simulink model "Ass2_Full"  (R2024b)
settings: Solver=VariableStepAuto  StartTime=0.0  StopTime=0.3  MaxStep=1e-5  RelTol=1e-4
values from neighbouring files (symbols this model uses):
  Cdc = 2*tau_C*Sn_n1/Vdcref_n1^2    (= 0.277777777778)    [PMSG_B2B_init.m]
  Rs = 0.01    [PMSG_B2B_init.m]
undefined symbols (not defined in the file or in its folder): a, f, G, Gn, Gstep, idref, iqref, Isc, Ki, kic, kip, kiv, kpc, kpp, kpv, Kv, L, Lg, par, Pref, Qref, Rc, Rg, Rp, ser, T, Tn, Tstep, Vdc_ref, Voc, Vpeak, Vt
libraries: spsControlledVoltageSourceLib x6, slpidlib x6, spsVoltageMeasurementLib x4, spsControlledCurrentSourceLib x2, spsThreePhaseSeriesRLCBranchLib x2, spsCurrentMeasurementLib x2, spsGroundLib x2, spsThreePhaseVIMeasurementLib x1, spsSeriesRLCBranchLib x1, sps_lib x1
settings Model: Creator=sproj  LastModifiedBy=sproj

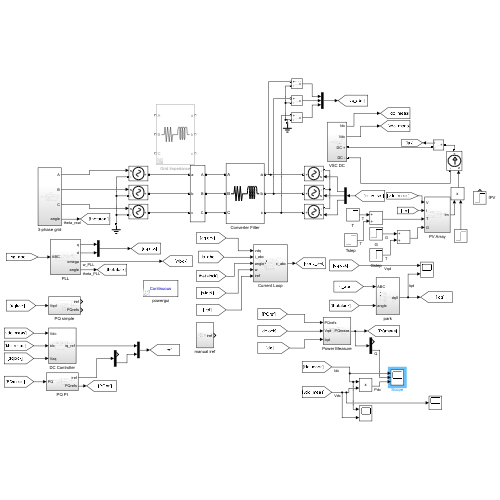
[thumbnail: Simulink's stored preview of the top-level diagram]
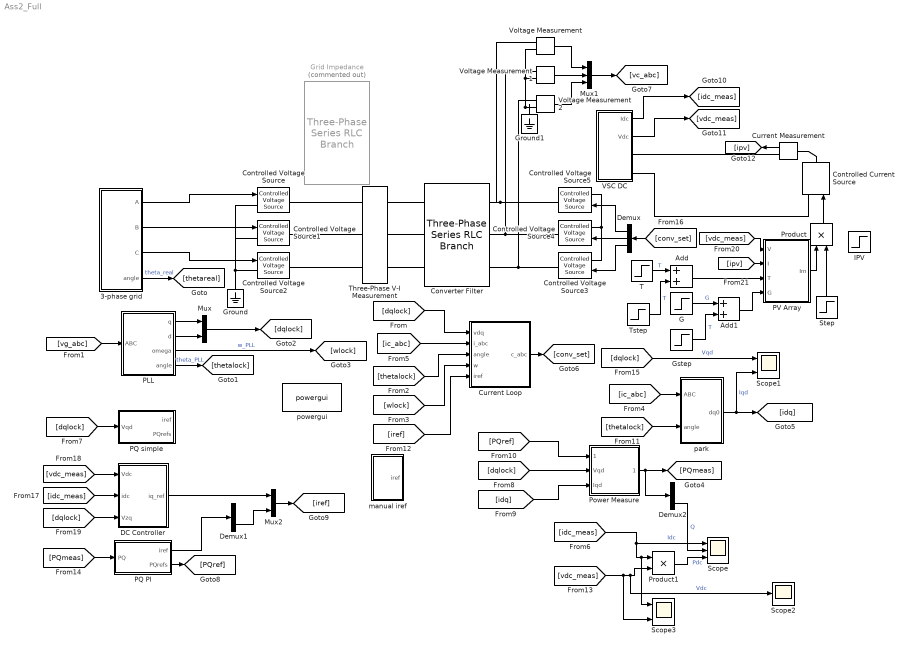
== system Ass2_Full ==
  3-phase grid : Subsystem
  Add : Sum
  Add1 : Sum
  Controlled Current Source : spsControlledCurrentSourceLib/Controlled Current Source  Initialize=on  Source_Type=AC  Amplitude=0  Phase=0  Frequency=0  Measurements=None
  Controlled Voltage Source{,1..5} (6 alike) : spsControlledVoltageSourceLib/Controlled Voltage Source  Initialize=on  Source_Type=AC  Amplitude=0  Phase=0  Frequency=0  Measurements=None
  Converter Filter : spsThreePhaseSeriesRLCBranchLib/Three-Phase Series RLC Branch  LConnTagsString=A|B|C  RConnTagsString=A|B|C  BranchType=RL  Resistance=Rc  Inductance=L  Capacitance=1e-6  Measurements=None
  Current Loop : Subsystem
  Current Measurement : spsCurrentMeasurementLib/Current Measurement  PhasorSimulation=off  OutputType=Complex  PSBequivalent=0
  DC Controller : Subsystem
  Demux : Demux  Outputs=3
  Demux1 : Demux  Outputs=2
  Demux2 : Demux  Outputs=2
  G : Step  Time=0  After=G  SampleTime=0
  Grid Impedance : spsThreePhaseSeriesRLCBranchLib/Three-Phase Series RLC Branch  Commented=on  LConnTagsString=A|B|C  RConnTagsString=A|B|C  BranchType=RL  Resistance=Rg  Inductance=Lg  Capacitance=1e-6  Measurements=None
  Ground : spsGroundLib/Ground  LConnTagsString=a
  Ground1 : spsGroundLib/Ground  LConnTagsString=a
  Gstep : Step  Time=0.05  After=Gstep  SampleTime=0
  IPV : Step  Time=0.1  After=4000  SampleTime=0
  Mux : Mux  Inputs=2
  Mux1 : Mux  Inputs=3
  Mux2 : Mux  Inputs=2
  PLL : Subsystem
  PQ PI : Subsystem
  PQ simple : Subsystem
  PV Array : Subsystem
  Power Measure : Subsystem
  Product : Product
  Product1 : Product
  Scope : Scope  NumInputPorts=3
  Scope1 : Scope  NumInputPorts=2
  Scope2 : Scope
  Scope3 : Scope  NumInputPorts=2
  Step : Step  Time=0.01  SampleTime=0
  T : Step  Time=0  After=T  SampleTime=0
  Three-Phase V-I Measurement : spsThreePhaseVIMeasurementLib/Three-Phase V-I Measurement  VoltageMeasurement=phase-to-ground  SetLabelV=on  LabelV=vg_abc  Vpu=off  VpuLL=off  CurrentMeasurement=yes  SetLabelI=on  LabelI=ic_abc  Ipu=off  Pbase=100e6  Vbase=500e3  OutputType=Complex  PhasorSimulation=off  PSBequivalent=0
  Tstep : Step  Time=0.05  After=Tstep  SampleTime=0
  VSC DC : Subsystem
  Voltage Measurement : spsVoltageMeasurementLib/Voltage Measurement  PhasorSimulation=off  OutputType=Complex  PSBequivalent=0
  Voltage Measurement1 : spsVoltageMeasurementLib/Voltage Measurement  PhasorSimulation=off  OutputType=Complex  PSBequivalent=0
  Voltage Measurement2 : spsVoltageMeasurementLib/Voltage Measurement  PhasorSimulation=off  OutputType=Complex  PSBequivalent=0
  manual iref : Subsystem
  park : Subsystem
  powergui : sps_lib/powergui  Priority=1  SimulationMode=Continuous  SampleTime=50e-6  frequency=60  Iterations=50  frequencyindice=0  Pbase=100e6  ErrMax=1e-4  UnitsV=kV  UnitsW=MW  buscounter=0  FunctionMessages=off  echomessages=off  EnableUseOfTLC=off  CurrentSourceSwitches=off  DisableSnubberDevices=off  DisableRonSwitches=off  DisableVfSwitches=off  DisplayEquations=off  AutomaticDiscreteSolvers=off  SolverType=Tustin/Backward Euler (TBE)  Interpol=off  ExternalGateDelay=off  methode=off  Ts=100  x0status=blocks  SPID=on  SwTol=0  HookPort=off  NonlinearTolerance=1e-4  nMaxIteration=100  ContinueOnMaxIteration=off  RestoreLinks=warning  ResistiveCurrentMeasurement=off  Frange=[0:2:500]  Ylog=off  Xlog=on  ShowGrid=off  save=off  variable=ZData  structure=0  ZoomFFT=off  StartTime=0.0  cycles=1  DisplayStyle=1  fundamental=60  FreqAxis=off  MaxFrequency=1000  frequencyindicesteady=1  RmsSteady=1  display=off
  wires:
  3-phase grid/1(A) -> Controlled Voltage Source/1
  3-phase grid/3(C) -> Controlled Voltage Source2/1
  3-phase grid/4(angle) -> [thetareal]  "theta_real"
  [vg_abc] -> PLL/1(ABC)
  PLL/4(angle) -> [thetalock]  "theta_PLL"
  PLL/1(q) -> Mux/1
  PLL/2(d) -> Mux/2
  Mux/1 -> [dqlock]
  PLL/3(omega) -> [wlock]  "w_PLL"
  [dqlock] -> Current Loop/1(vdq)
  [ic_abc] -> Current Loop/2(i_abc)
  [thetalock] -> Current Loop/3(angle)
  [wlock] -> Current Loop/4(w)
  [ic_abc] -> park/1(ABC)
  [dqlock] -> PQ simple/1(Vqd)
  [PQref] -> Power Measure/1(PQrefs)
  [dqlock] -> Power Measure/2(Vqd)
  [idq] -> Power Measure/3(Iqd)
  [thetalock] -> park/2(angle)
  [iref] -> Current Loop/5(iref)
  Voltage Measurement1/1 -> Mux1/2
  Voltage Measurement/1 -> Mux1/1
  Voltage Measurement2/1 -> Mux1/3
  Mux1/1 -> [vc_abc]
  3-phase grid/2(B) -> Controlled Voltage Source1/1
  [vdc_meas] -> Scope3/2, Scope2/1, Product1/2  "Vdc"
  Power Measure/1(PQmeas) -> Demux2/1, [PQmeas]
  [PQmeas] -> PQ PI/1(PQ)
  park/1(dq0) -> Scope1/2, [idq]  "Iqd"
  [dqlock] -> Scope1/1  "Vqd"
  PQ PI/2(PQrefs) -> [PQref]
  Current Loop/1(c_abc) -> [conv_set]
  [conv_set] -> Demux/1
  Demux/1 -> Controlled Voltage Source5/1
  Demux/2 -> Controlled Voltage Source4/1
  Demux/3 -> Controlled Voltage Source3/1
  PQ PI/1(iref) -> Demux1/1
  Mux2/1 -> [iref]
  DC Controller/1(iq_ref) -> Mux2/1
  Demux1/2 -> Mux2/2
  [idc_meas] -> DC Controller/2(idc)
  VSC DC/2(Vdc) -> [vdc_meas]
  [vdc_meas] -> DC Controller/1(Vdc)
  [dqlock] -> DC Controller/3(Vzq)
  VSC DC/1(Idc) -> [idc_meas]
  [vdc_meas] -> PV Array/1(V)
  Current Measurement/1 -> [ipv]
  [ipv] -> PV Array/2(I)
  Step/1 -> Product/2
  PV Array/1(Im) -> Product/1
  [idc_meas] -> Scope3/1, Product1/1, Scope/1  "Idc"
  T/1 -> Add/1  "T"
  Tstep/1 -> Add/2  "T"
  Add/1 -> PV Array/3(T)
  G/1 -> Add1/1  "G"
  Gstep/1 -> Add1/2  "T"
  Add1/1 -> PV Array/4(G)
  Demux2/2 -> Scope/2  "Q"
  Product1/1 -> Scope/3  "Pdc"
  Product/1 -> Controlled Current Source/1
  connections:
  Ground/LConn1 -- Controlled Voltage Source/LConn1 -- Controlled Voltage Source1/LConn1 -- Controlled Voltage Source2/LConn1
  Controlled Voltage Source5/LConn1 -- Controlled Voltage Source3/LConn1 -- Controlled Voltage Source4/LConn1
  Converter Filter/RConn3 -- Controlled Voltage Source3/RConn1 -- Voltage Measurement2/LConn1
  Converter Filter/RConn2 -- Controlled Voltage Source4/RConn1 -- Voltage Measurement1/LConn1
  Converter Filter/RConn1 -- Controlled Voltage Source5/RConn1 -- Voltage Measurement/LConn1
  Voltage Measurement2/LConn2 -- Ground1/LConn1 -- Voltage Measurement/LConn2 -- Voltage Measurement1/LConn2
  Three-Phase V-I Measurement/LConn1 -- Converter Filter/LConn1
  Three-Phase V-I Measurement/LConn2 -- Converter Filter/LConn2
  Three-Phase V-I Measurement/LConn3 -- Converter Filter/LConn3
  Controlled Voltage Source1/RConn1 -- Three-Phase V-I Measurement/RConn2
  Controlled Voltage Source2/RConn1 -- Three-Phase V-I Measurement/RConn3
  Three-Phase V-I Measurement/RConn1 -- Controlled Voltage Source/RConn1
  Controlled Current Source/LConn1 -- VSC DC/RConn2
  Current Measurement/LConn1 -- Controlled Current Source/RConn1
  Current Measurement/RConn1 -- VSC DC/RConn1

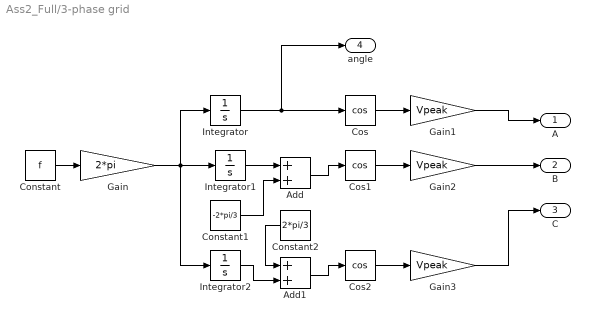
== system Ass2_Full/3-phase grid ==
  Add : Sum
  Add1 : Sum
  Constant : Constant  Value=f
  Constant1 : Constant  Value=-2*pi/3
  Constant2 : Constant  Value=2*pi/3
  Cos : Trigonometry  Operator=cos
  Cos1 : Trigonometry  Operator=cos
  Cos2 : Trigonometry  Operator=cos
  Gain : Gain  Gain=2*pi
  Gain1 : Gain  Gain=Vpeak
  Gain2 : Gain  Gain=Vpeak
  Gain3 : Gain  Gain=Vpeak
  Integrator : Integrator
  Integrator1 : Integrator
  Integrator2 : Integrator
  A : Outport
  B : Outport  Port=2
  C : Outport  Port=3
  angle : Outport  Port=4
  wires:
  Constant1/1 -> Add/2
  Cos2/1 -> Gain3/1
  Integrator1/1 -> Add/1
  Cos/1 -> Gain1/1
  Constant/1 -> Gain/1
  Add/1 -> Cos1/1
  Gain/1 -> Integrator2/1, Integrator/1, Integrator1/1
  Cos1/1 -> Gain2/1
  Add1/1 -> Cos2/1
  Integrator/1 -> angle/1, Cos/1
  Gain3/1 -> C/1
  Gain1/1 -> A/1
  Gain2/1 -> B/1
  Constant2/1 -> Add1/1
  Integrator2/1 -> Add1/2

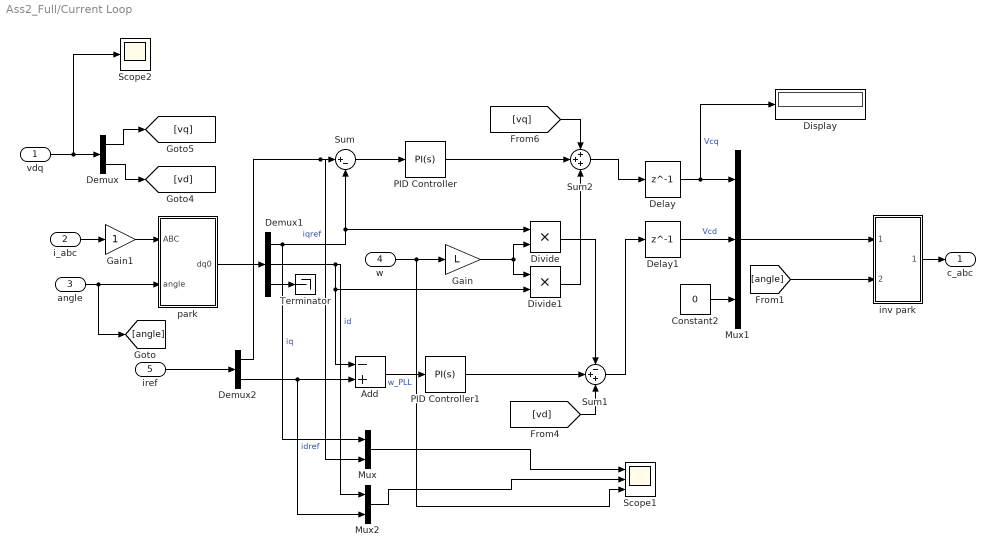
== system Ass2_Full/Current Loop ==
  vdq : Inport
  i_abc : Inport  Port=2
  angle : Inport  Port=3
  w : Inport  Port=4
  iref : Inport  Port=5
  Add : Sum  Inputs=-+
  Constant2 : Constant  Value=0
  Delay : Delay  DelayLength=1  InputProcessing=Columns as channels (frame based)
  Delay1 : Delay  DelayLength=1  InputProcessing=Columns as channels (frame based)
  Demux : Demux  Outputs=2
  Demux1 : Demux  Outputs=3
  Demux2 : Demux  Outputs=2
  Display : Display
  Divide : Product
  Divide1 : Product
  Gain : Gain  Gain=L
  Gain1 : Gain
  Mux : Mux  Inputs=2
  Mux1 : Mux  Inputs=3
  Mux2 : Mux  Inputs=2
  PID Controller : slpidlib/PID Controller  Controller=PI  Form=Parallel  TimeDomain=Continuous-time  UseExternalTs=off  SampleTime=-1  IntegratorMethod=Forward Euler  FilterMethod=Forward Euler  ControllerParametersSource=internal  P=kpc  I=kic  UseKiTs=off  D=0  UseExternalDerivativeSource=off  N=100  UseFilter=on  TunerSelectOption=Transfer Function Based (PID Tuner App)  InitialConditionSource=internal  InitialConditionForIntegrator=0  InitialConditionForFilter=0  DifferentiatorICPrevScaledInput=0  ExternalReset=none  TrackingMode=off  Kt=1  LimitOutput=off  SatLimitsSource=internal  UpperSaturationLimit=inf  LowerSaturationLimit=-inf  LinearizeAsGain=on  AntiWindupMode=none  Kb=1  LimitIntegrator=off  UpperIntegratorSaturationLimit=inf  LowerIntegratorSaturationLimit=-inf  POutMin=[]  POutMax=[]  IOutMin=[]  IOutMax=[]  DOutMin=[]  DOutMax=[]  NOutMin=[]  NOutMax=[]  SumOutMin=[]  SumOutMax=[]  SaturationOutMin=[]  SaturationOutMax=[]  PParamMin=[]  PParamMax=[]  IParamMin=[]  IParamMax=[]  DParamMin=[]  DParamMax=[]  NParamMin=[]  NParamMax=[]  KbParamMin=[]  KbParamMax=[]  KtParamMin=[]  KtParamMax=[]  KbOutMin=[]  KbOutMax=[]  KtOutMin=[]  KtOutMax=[]  IntegratorOutMin=[]  IntegratorOutMax=[]  FilterOutMin=[]  FilterOutMax=[]  SumI1OutMin=[]  SumI1OutMax=[]  SumI2OutMin=[]  SumI2OutMax=[]  SumI3OutMin=[]  SumI3OutMax=[]  SumI4OutMin=[]  SumI4OutMax=[]  SumDOutMin=[]  SumDOutMax=[]  DifferentiatorOutMin=[]  DifferentiatorOutMax=[]  FilterDiffOutCoefMin=[]  FilterDiffOutCoefMax=[]  ReciprocalOutMin=[]  ReciprocalOutMax=[]  SumDenOutMin=[]  SumDenOutMax=[]  SumNumOutMin=[]  SumNumOutMax=[]  DivideOutMin=[]  DivideOutMax=[]  UdiffTsProdOutMin=[]  UdiffTsProdOutMax=[]  NTsProdOutMin=[]  NTsProdOutMax=[]  UintegralTsProdOutMin=[]  UintegralTsProdOutMax=[]  UngainTsProdOutMin=[]  UngainTsProdOutMax=[]  ClampingZeroOutDataTypeStr=Inherit: Inherit via back propagation  ClampingZeroOutMin=[]  ClampingZeroOutMax=[]  FilterDenConstantOutDataTypeStr=Inherit: Inherit via back propagation  FilterDenConstantOutMin=[]  FilterDenConstantOutMax=[]  PCopyOutDataTypeStr=Inherit: Inherit via back propagation  PCopyOutMin=[]  PCopyOutMax=[]  NCopyOutDataTypeStr=Inherit: Inherit via back propagation  NCopyOutMin=[]  NCopyOutMax=[]  IntegratorContinuousStateAttributes=''  IntegratorStateMustResolveToSignalObject=off  IntegratorRTWStateStorageClass=Auto  FilterContinuousStateAttributes=''  FilterStateMustResolveToSignalObject=off  FilterRTWStateStorageClass=Auto  ParallelPVariant=InternalParameters  IdealPVariant=Disabled  IVariant=InternalParameters  DVariant=Disabled  IntegratorVariant=Continuous  SatVariant=Disabled  AWVariant=Passthrough  PCopyVariant=Disabled  TRVariant=Disabled  FdbkBlocksVariant=Forward  IdealPFdbkVariant=Disabled  SatFdbkVariant=Disabled  DerivativeFilterVariant=Disabled  NVariant=Disabled  NCopyVariant=Disabled_SignalSpec  FilterICVariant=Disabled  IntegratorICVariant=InternalICs  ExternalResetVariant=Disabled  TRSumVariant=Passthrough  SumFdbkVariant=Disabled  SumVariant=Sum_PI  TsampFilterVariant=InternalTs  TsampNgainVariant=Passthrough  TsampIntegralVariant=Disabled_SignalSpec  ExternalSaturationOutDataTypeStr=Inherit: Same as second input  DerivativeSourceVariant=Disabled  PreIntVariant=InternalPreInt
  PID Controller1 : slpidlib/PID Controller  Controller=PI  Form=Parallel  TimeDomain=Continuous-time  UseExternalTs=off  SampleTime=-1  IntegratorMethod=Forward Euler  FilterMethod=Forward Euler  ControllerParametersSource=internal  P=kpc  I=kic  UseKiTs=off  D=0  UseExternalDerivativeSource=off  N=100  UseFilter=on  TunerSelectOption=Transfer Function Based (PID Tuner App)  InitialConditionSource=internal  InitialConditionForIntegrator=0  InitialConditionForFilter=0  DifferentiatorICPrevScaledInput=0  ExternalReset=none  TrackingMode=off  Kt=1  LimitOutput=off  SatLimitsSource=internal  UpperSaturationLimit=inf  LowerSaturationLimit=-inf  LinearizeAsGain=on  AntiWindupMode=none  Kb=1  LimitIntegrator=off  UpperIntegratorSaturationLimit=inf  LowerIntegratorSaturationLimit=-inf  POutMin=[]  POutMax=[]  IOutMin=[]  IOutMax=[]  DOutMin=[]  DOutMax=[]  NOutMin=[]  NOutMax=[]  SumOutMin=[]  SumOutMax=[]  SaturationOutMin=[]  SaturationOutMax=[]  PParamMin=[]  PParamMax=[]  IParamMin=[]  IParamMax=[]  DParamMin=[]  DParamMax=[]  NParamMin=[]  NParamMax=[]  KbParamMin=[]  KbParamMax=[]  KtParamMin=[]  KtParamMax=[]  KbOutMin=[]  KbOutMax=[]  KtOutMin=[]  KtOutMax=[]  IntegratorOutMin=[]  IntegratorOutMax=[]  FilterOutMin=[]  FilterOutMax=[]  SumI1OutMin=[]  SumI1OutMax=[]  SumI2OutMin=[]  SumI2OutMax=[]  SumI3OutMin=[]  SumI3OutMax=[]  SumI4OutMin=[]  SumI4OutMax=[]  SumDOutMin=[]  SumDOutMax=[]  DifferentiatorOutMin=[]  DifferentiatorOutMax=[]  FilterDiffOutCoefMin=[]  FilterDiffOutCoefMax=[]  ReciprocalOutMin=[]  ReciprocalOutMax=[]  SumDenOutMin=[]  SumDenOutMax=[]  SumNumOutMin=[]  SumNumOutMax=[]  DivideOutMin=[]  DivideOutMax=[]  UdiffTsProdOutMin=[]  UdiffTsProdOutMax=[]  NTsProdOutMin=[]  NTsProdOutMax=[]  UintegralTsProdOutMin=[]  UintegralTsProdOutMax=[]  UngainTsProdOutMin=[]  UngainTsProdOutMax=[]  ClampingZeroOutDataTypeStr=Inherit: Inherit via back propagation  ClampingZeroOutMin=[]  ClampingZeroOutMax=[]  FilterDenConstantOutDataTypeStr=Inherit: Inherit via back propagation  FilterDenConstantOutMin=[]  FilterDenConstantOutMax=[]  PCopyOutDataTypeStr=Inherit: Inherit via back propagation  PCopyOutMin=[]  PCopyOutMax=[]  NCopyOutDataTypeStr=Inherit: Inherit via back propagation  NCopyOutMin=[]  NCopyOutMax=[]  IntegratorContinuousStateAttributes=''  IntegratorStateMustResolveToSignalObject=off  IntegratorRTWStateStorageClass=Auto  FilterContinuousStateAttributes=''  FilterStateMustResolveToSignalObject=off  FilterRTWStateStorageClass=Auto  ParallelPVariant=InternalParameters  IdealPVariant=Disabled  IVariant=InternalParameters  DVariant=Disabled  IntegratorVariant=Continuous  SatVariant=Disabled  AWVariant=Passthrough  PCopyVariant=Disabled  TRVariant=Disabled  FdbkBlocksVariant=Forward  IdealPFdbkVariant=Disabled  SatFdbkVariant=Disabled  DerivativeFilterVariant=Disabled  NVariant=Disabled  NCopyVariant=Disabled_SignalSpec  FilterICVariant=Disabled  IntegratorICVariant=InternalICs  ExternalResetVariant=Disabled  TRSumVariant=Passthrough  SumFdbkVariant=Disabled  SumVariant=Sum_PI  TsampFilterVariant=InternalTs  TsampNgainVariant=Passthrough  TsampIntegralVariant=Disabled_SignalSpec  ExternalSaturationOutDataTypeStr=Inherit: Same as second input  DerivativeSourceVariant=Disabled  PreIntVariant=InternalPreInt
  Scope1 : Scope  NumInputPorts=3
  Scope2 : Scope
  Sum : Sum  Inputs=|+-
  Sum1 : Sum  Inputs=-++
  Sum2 : Sum  Inputs=+++
  Terminator : Terminator
  inv park : Subsystem
  park : Subsystem
  c_abc : Outport
  wires:
  PID Controller/1 -> Sum2/2
  Demux2/1 -> Mux/2, Sum/1  "iqref"
  angle/1 -> [angle], park/2(angle)
  Constant2/1 -> Mux1/3
  Demux1/3 -> Terminator/1
  Demux1/2 -> Mux2/1, Divide1/2, Add/1  "id"
  Divide/1 -> Sum1/1
  park/1(dq0) -> Demux1/1
  Demux2/2 -> Mux2/2, Add/2  "idref"
  Mux1/1 -> inv park/1(qd0)
  i_abc/1 -> Gain1/1
  vdq/1 -> Scope2/1, Demux/1
  Demux1/1 -> Mux/1, Divide/1, Sum/2  "iq"
  Sum/1 -> PID Controller/1
  Add/1 -> PID Controller1/1
  PID Controller1/1 -> Sum1/2
  Divide1/1 -> Sum2/3
  Gain/1 -> Divide1/1, Divide/2
  inv park/1(ABC) -> c_abc/1
  [angle] -> inv park/2(angle)
  Sum2/1 -> Delay/1
  Delay/1 -> Display/1, Mux1/1  "Vcq"
  Delay1/1 -> Mux1/2  "Vcd"
  Sum1/1 -> Delay1/1
  Gain1/1 -> park/1(ABC)
  [vq] -> Sum2/1
  Demux/1 -> [vq]
  Demux/2 -> [vd]
  [vd] -> Sum1/3
  iref/1 -> Demux2/1
  Mux/1 -> Scope1/1
  Mux2/1 -> Scope1/2
  w/1 -> Scope1/3, Gain/1  "w_PLL"

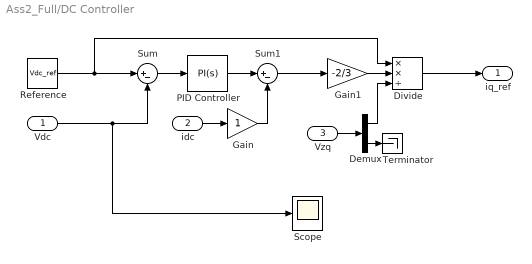
== system Ass2_Full/DC Controller ==
  Vdc : Inport
  idc : Inport  Port=2
  Vzq : Inport  Port=3
  Demux : Demux  Outputs=2
  Divide : Product  Inputs=**/
  Gain : Gain
  Gain1 : Gain  Gain=-2/3
  PID Controller : slpidlib/PID Controller  Controller=PI  Form=Parallel  TimeDomain=Continuous-time  UseExternalTs=off  SampleTime=-1  IntegratorMethod=Forward Euler  FilterMethod=Forward Euler  ControllerParametersSource=internal  P=kpv  I=kiv  UseKiTs=off  D=0  UseExternalDerivativeSource=off  N=100  UseFilter=on  TunerSelectOption=Transfer Function Based (PID Tuner App)  InitialConditionSource=internal  InitialConditionForIntegrator=0  InitialConditionForFilter=0  DifferentiatorICPrevScaledInput=0  ExternalReset=none  TrackingMode=off  Kt=1  LimitOutput=off  SatLimitsSource=internal  UpperSaturationLimit=inf  LowerSaturationLimit=-inf  LinearizeAsGain=on  AntiWindupMode=none  Kb=1  LimitIntegrator=off  UpperIntegratorSaturationLimit=inf  LowerIntegratorSaturationLimit=-inf  POutMin=[]  POutMax=[]  IOutMin=[]  IOutMax=[]  DOutMin=[]  DOutMax=[]  NOutMin=[]  NOutMax=[]  SumOutMin=[]  SumOutMax=[]  SaturationOutMin=[]  SaturationOutMax=[]  PParamMin=[]  PParamMax=[]  IParamMin=[]  IParamMax=[]  DParamMin=[]  DParamMax=[]  NParamMin=[]  NParamMax=[]  KbParamMin=[]  KbParamMax=[]  KtParamMin=[]  KtParamMax=[]  KbOutMin=[]  KbOutMax=[]  KtOutMin=[]  KtOutMax=[]  IntegratorOutMin=[]  IntegratorOutMax=[]  FilterOutMin=[]  FilterOutMax=[]  SumI1OutMin=[]  SumI1OutMax=[]  SumI2OutMin=[]  SumI2OutMax=[]  SumI3OutMin=[]  SumI3OutMax=[]  SumI4OutMin=[]  SumI4OutMax=[]  SumDOutMin=[]  SumDOutMax=[]  DifferentiatorOutMin=[]  DifferentiatorOutMax=[]  FilterDiffOutCoefMin=[]  FilterDiffOutCoefMax=[]  ReciprocalOutMin=[]  ReciprocalOutMax=[]  SumDenOutMin=[]  SumDenOutMax=[]  SumNumOutMin=[]  SumNumOutMax=[]  DivideOutMin=[]  DivideOutMax=[]  UdiffTsProdOutMin=[]  UdiffTsProdOutMax=[]  NTsProdOutMin=[]  NTsProdOutMax=[]  UintegralTsProdOutMin=[]  UintegralTsProdOutMax=[]  UngainTsProdOutMin=[]  UngainTsProdOutMax=[]  ClampingZeroOutDataTypeStr=Inherit: Inherit via back propagation  ClampingZeroOutMin=[]  ClampingZeroOutMax=[]  FilterDenConstantOutDataTypeStr=Inherit: Inherit via back propagation  FilterDenConstantOutMin=[]  FilterDenConstantOutMax=[]  PCopyOutDataTypeStr=Inherit: Inherit via back propagation  PCopyOutMin=[]  PCopyOutMax=[]  NCopyOutDataTypeStr=Inherit: Inherit via back propagation  NCopyOutMin=[]  NCopyOutMax=[]  IntegratorContinuousStateAttributes=''  IntegratorStateMustResolveToSignalObject=off  IntegratorRTWStateStorageClass=Auto  FilterContinuousStateAttributes=''  FilterStateMustResolveToSignalObject=off  FilterRTWStateStorageClass=Auto  ParallelPVariant=InternalParameters  IdealPVariant=Disabled  IVariant=InternalParameters  DVariant=Disabled  IntegratorVariant=Continuous  SatVariant=Disabled  AWVariant=Passthrough  PCopyVariant=Disabled  TRVariant=Disabled  FdbkBlocksVariant=Forward  IdealPFdbkVariant=Disabled  SatFdbkVariant=Disabled  DerivativeFilterVariant=Disabled  NVariant=Disabled  NCopyVariant=Disabled_SignalSpec  FilterICVariant=Disabled  IntegratorICVariant=InternalICs  ExternalResetVariant=Disabled  TRSumVariant=Passthrough  SumFdbkVariant=Disabled  SumVariant=Sum_PI  TsampFilterVariant=InternalTs  TsampNgainVariant=Passthrough  TsampIntegralVariant=Disabled_SignalSpec  ExternalSaturationOutDataTypeStr=Inherit: Same as second input  DerivativeSourceVariant=Disabled  PreIntVariant=InternalPreInt
  Reference : Constant  Value=Vdc_ref
  Scope : Scope
  Sum : Sum  Inputs=|+-
  Sum1 : Sum  Inputs=|+-
  Terminator : Terminator
  iq_ref : Outport
  wires:
  Sum/1 -> PID Controller/1
  Sum1/1 -> Gain1/1
  Reference/1 -> Divide/1, Sum/1
  PID Controller/1 -> Sum1/1
  idc/1 -> Gain/1
  Vdc/1 -> Scope/1, Sum/2
  Gain1/1 -> Divide/2
  Gain/1 -> Sum1/2
  Divide/1 -> iq_ref/1
  Vzq/1 -> Demux/1
  Demux/1 -> Divide/3
  Demux/2 -> Terminator/1

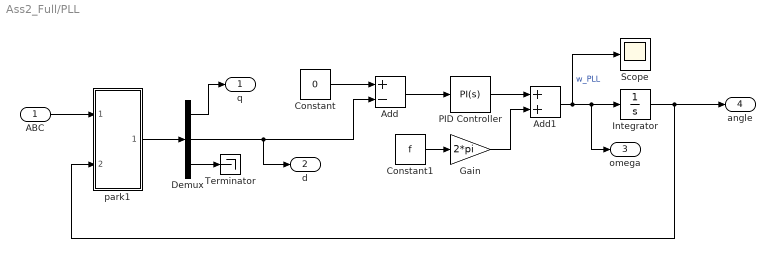
== system Ass2_Full/PLL ==
  ABC : Inport
  Add : Sum  Inputs=+-
  Add1 : Sum
  Constant : Constant  Value=0
  Constant1 : Constant  Value=f
  Demux : Demux  Outputs=3
  Gain : Gain  Gain=2*pi
  Integrator : Integrator
  PID Controller : slpidlib/PID Controller  Controller=PI  Form=Parallel  TimeDomain=Continuous-time  UseExternalTs=off  SampleTime=-1  IntegratorMethod=Forward Euler  FilterMethod=Forward Euler  ControllerParametersSource=internal  P=0.78849  I=175.18  UseKiTs=off  D=0  UseExternalDerivativeSource=off  N=100  UseFilter=on  TunerSelectOption=Transfer Function Based (PID Tuner App)  InitialConditionSource=internal  InitialConditionForIntegrator=0  InitialConditionForFilter=0  DifferentiatorICPrevScaledInput=0  ExternalReset=none  TrackingMode=off  Kt=1  LimitOutput=off  SatLimitsSource=internal  UpperSaturationLimit=inf  LowerSaturationLimit=-inf  LinearizeAsGain=on  AntiWindupMode=none  Kb=1  LimitIntegrator=off  UpperIntegratorSaturationLimit=inf  LowerIntegratorSaturationLimit=-inf  POutMin=[]  POutMax=[]  IOutMin=[]  IOutMax=[]  DOutMin=[]  DOutMax=[]  NOutMin=[]  NOutMax=[]  SumOutMin=[]  SumOutMax=[]  SaturationOutMin=[]  SaturationOutMax=[]  PParamMin=[]  PParamMax=[]  IParamMin=[]  IParamMax=[]  DParamMin=[]  DParamMax=[]  NParamMin=[]  NParamMax=[]  KbParamMin=[]  KbParamMax=[]  KtParamMin=[]  KtParamMax=[]  KbOutMin=[]  KbOutMax=[]  KtOutMin=[]  KtOutMax=[]  IntegratorOutMin=[]  IntegratorOutMax=[]  FilterOutMin=[]  FilterOutMax=[]  SumI1OutMin=[]  SumI1OutMax=[]  SumI2OutMin=[]  SumI2OutMax=[]  SumI3OutMin=[]  SumI3OutMax=[]  SumI4OutMin=[]  SumI4OutMax=[]  SumDOutMin=[]  SumDOutMax=[]  DifferentiatorOutMin=[]  DifferentiatorOutMax=[]  FilterDiffOutCoefMin=[]  FilterDiffOutCoefMax=[]  ReciprocalOutMin=[]  ReciprocalOutMax=[]  SumDenOutMin=[]  SumDenOutMax=[]  SumNumOutMin=[]  SumNumOutMax=[]  DivideOutMin=[]  DivideOutMax=[]  UdiffTsProdOutMin=[]  UdiffTsProdOutMax=[]  NTsProdOutMin=[]  NTsProdOutMax=[]  UintegralTsProdOutMin=[]  UintegralTsProdOutMax=[]  UngainTsProdOutMin=[]  UngainTsProdOutMax=[]  ClampingZeroOutDataTypeStr=Inherit: Inherit via back propagation  ClampingZeroOutMin=[]  ClampingZeroOutMax=[]  FilterDenConstantOutDataTypeStr=Inherit: Inherit via back propagation  FilterDenConstantOutMin=[]  FilterDenConstantOutMax=[]  PCopyOutDataTypeStr=Inherit: Inherit via back propagation  PCopyOutMin=[]  PCopyOutMax=[]  NCopyOutDataTypeStr=Inherit: Inherit via back propagation  NCopyOutMin=[]  NCopyOutMax=[]  IntegratorContinuousStateAttributes=''  IntegratorStateMustResolveToSignalObject=off  IntegratorRTWStateStorageClass=Auto  FilterContinuousStateAttributes=''  FilterStateMustResolveToSignalObject=off  FilterRTWStateStorageClass=Auto  ParallelPVariant=InternalParameters  IdealPVariant=Disabled  IVariant=InternalParameters  DVariant=Disabled  IntegratorVariant=Continuous  SatVariant=Disabled  AWVariant=Passthrough  PCopyVariant=Disabled  TRVariant=Disabled  FdbkBlocksVariant=Forward  IdealPFdbkVariant=Disabled  SatFdbkVariant=Disabled  DerivativeFilterVariant=Disabled  NVariant=Disabled  NCopyVariant=Disabled_SignalSpec  FilterICVariant=Disabled  IntegratorICVariant=InternalICs  ExternalResetVariant=Disabled  TRSumVariant=Passthrough  SumFdbkVariant=Disabled  SumVariant=Sum_PI  TsampFilterVariant=InternalTs  TsampNgainVariant=Passthrough  TsampIntegralVariant=Disabled_SignalSpec  ExternalSaturationOutDataTypeStr=Inherit: Same as second input  DerivativeSourceVariant=Disabled  PreIntVariant=InternalPreInt
  Scope : Scope
  Terminator : Terminator
  park1 : Subsystem
  q : Outport
  d : Outport  Port=2
  omega : Outport  Port=3
  angle : Outport  Port=4
  wires:
  Demux/3 -> Terminator/1
  Add1/1 -> Scope/1, omega/1, Integrator/1  "w_PLL"
  Gain/1 -> Add1/2
  park1/1(dq0) -> Demux/1
  Constant1/1 -> Gain/1
  Demux/2 -> d/1, Add/2
  Constant/1 -> Add/1
  Add/1 -> PID Controller/1
  Integrator/1 -> angle/1, park1/2(angle)
  Demux/1 -> q/1
  PID Controller/1 -> Add1/1
  ABC/1 -> park1/1(ABC)

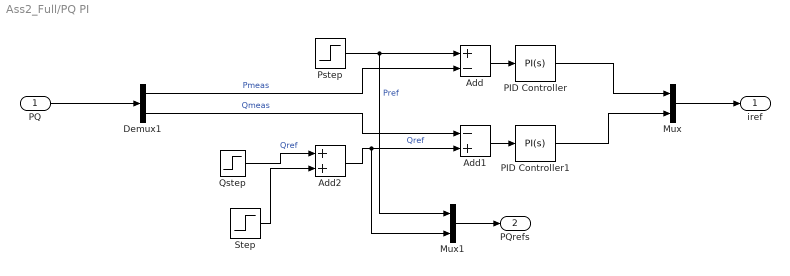
== system Ass2_Full/PQ PI ==
  PQ : Inport
  Add : Sum  Inputs=+-
  Add1 : Sum  Inputs=-+
  Add2 : Sum
  Demux1 : Demux  Outputs=2
  Mux : Mux  Inputs=2
  Mux1 : Mux  Inputs=2
  PID Controller : slpidlib/PID Controller  Controller=PI  Form=Parallel  TimeDomain=Continuous-time  UseExternalTs=off  SampleTime=-1  IntegratorMethod=Forward Euler  FilterMethod=Forward Euler  ControllerParametersSource=internal  P=kpp  I=kip  UseKiTs=off  D=0  UseExternalDerivativeSource=off  N=100  UseFilter=on  TunerSelectOption=Transfer Function Based (PID Tuner App)  InitialConditionSource=internal  InitialConditionForIntegrator=0  InitialConditionForFilter=0  DifferentiatorICPrevScaledInput=0  ExternalReset=none  TrackingMode=off  Kt=1  LimitOutput=off  SatLimitsSource=internal  UpperSaturationLimit=inf  LowerSaturationLimit=-inf  LinearizeAsGain=on  AntiWindupMode=none  Kb=1  LimitIntegrator=off  UpperIntegratorSaturationLimit=inf  LowerIntegratorSaturationLimit=-inf  POutMin=[]  POutMax=[]  IOutMin=[]  IOutMax=[]  DOutMin=[]  DOutMax=[]  NOutMin=[]  NOutMax=[]  SumOutMin=[]  SumOutMax=[]  SaturationOutMin=[]  SaturationOutMax=[]  PParamMin=[]  PParamMax=[]  IParamMin=[]  IParamMax=[]  DParamMin=[]  DParamMax=[]  NParamMin=[]  NParamMax=[]  KbParamMin=[]  KbParamMax=[]  KtParamMin=[]  KtParamMax=[]  KbOutMin=[]  KbOutMax=[]  KtOutMin=[]  KtOutMax=[]  IntegratorOutMin=[]  IntegratorOutMax=[]  FilterOutMin=[]  FilterOutMax=[]  SumI1OutMin=[]  SumI1OutMax=[]  SumI2OutMin=[]  SumI2OutMax=[]  SumI3OutMin=[]  SumI3OutMax=[]  SumI4OutMin=[]  SumI4OutMax=[]  SumDOutMin=[]  SumDOutMax=[]  DifferentiatorOutMin=[]  DifferentiatorOutMax=[]  FilterDiffOutCoefMin=[]  FilterDiffOutCoefMax=[]  ReciprocalOutMin=[]  ReciprocalOutMax=[]  SumDenOutMin=[]  SumDenOutMax=[]  SumNumOutMin=[]  SumNumOutMax=[]  DivideOutMin=[]  DivideOutMax=[]  UdiffTsProdOutMin=[]  UdiffTsProdOutMax=[]  NTsProdOutMin=[]  NTsProdOutMax=[]  UintegralTsProdOutMin=[]  UintegralTsProdOutMax=[]  UngainTsProdOutMin=[]  UngainTsProdOutMax=[]  ClampingZeroOutDataTypeStr=Inherit: Inherit via back propagation  ClampingZeroOutMin=[]  ClampingZeroOutMax=[]  FilterDenConstantOutDataTypeStr=Inherit: Inherit via back propagation  FilterDenConstantOutMin=[]  FilterDenConstantOutMax=[]  PCopyOutDataTypeStr=Inherit: Inherit via back propagation  PCopyOutMin=[]  PCopyOutMax=[]  NCopyOutDataTypeStr=Inherit: Inherit via back propagation  NCopyOutMin=[]  NCopyOutMax=[]  IntegratorContinuousStateAttributes=''  IntegratorStateMustResolveToSignalObject=off  IntegratorRTWStateStorageClass=Auto  FilterContinuousStateAttributes=''  FilterStateMustResolveToSignalObject=off  FilterRTWStateStorageClass=Auto  ParallelPVariant=InternalParameters  IdealPVariant=Disabled  IVariant=InternalParameters  DVariant=Disabled  IntegratorVariant=Continuous  SatVariant=Disabled  AWVariant=Passthrough  PCopyVariant=Disabled  TRVariant=Disabled  FdbkBlocksVariant=Forward  IdealPFdbkVariant=Disabled  SatFdbkVariant=Disabled  DerivativeFilterVariant=Disabled  NVariant=Disabled  NCopyVariant=Disabled_SignalSpec  FilterICVariant=Disabled  IntegratorICVariant=InternalICs  ExternalResetVariant=Disabled  TRSumVariant=Passthrough  SumFdbkVariant=Disabled  SumVariant=Sum_PI  TsampFilterVariant=InternalTs  TsampNgainVariant=Passthrough  TsampIntegralVariant=Disabled_SignalSpec  ExternalSaturationOutDataTypeStr=Inherit: Same as second input  DerivativeSourceVariant=Disabled  PreIntVariant=InternalPreInt
  PID Controller1 : slpidlib/PID Controller  Controller=PI  Form=Parallel  TimeDomain=Continuous-time  UseExternalTs=off  SampleTime=-1  IntegratorMethod=Forward Euler  FilterMethod=Forward Euler  ControllerParametersSource=internal  P=kpp  I=kip  UseKiTs=off  D=0  UseExternalDerivativeSource=off  N=100  UseFilter=on  TunerSelectOption=Transfer Function Based (PID Tuner App)  InitialConditionSource=internal  InitialConditionForIntegrator=0  InitialConditionForFilter=0  DifferentiatorICPrevScaledInput=0  ExternalReset=none  TrackingMode=off  Kt=1  LimitOutput=off  SatLimitsSource=internal  UpperSaturationLimit=inf  LowerSaturationLimit=-inf  LinearizeAsGain=on  AntiWindupMode=none  Kb=1  LimitIntegrator=off  UpperIntegratorSaturationLimit=inf  LowerIntegratorSaturationLimit=-inf  POutMin=[]  POutMax=[]  IOutMin=[]  IOutMax=[]  DOutMin=[]  DOutMax=[]  NOutMin=[]  NOutMax=[]  SumOutMin=[]  SumOutMax=[]  SaturationOutMin=[]  SaturationOutMax=[]  PParamMin=[]  PParamMax=[]  IParamMin=[]  IParamMax=[]  DParamMin=[]  DParamMax=[]  NParamMin=[]  NParamMax=[]  KbParamMin=[]  KbParamMax=[]  KtParamMin=[]  KtParamMax=[]  KbOutMin=[]  KbOutMax=[]  KtOutMin=[]  KtOutMax=[]  IntegratorOutMin=[]  IntegratorOutMax=[]  FilterOutMin=[]  FilterOutMax=[]  SumI1OutMin=[]  SumI1OutMax=[]  SumI2OutMin=[]  SumI2OutMax=[]  SumI3OutMin=[]  SumI3OutMax=[]  SumI4OutMin=[]  SumI4OutMax=[]  SumDOutMin=[]  SumDOutMax=[]  DifferentiatorOutMin=[]  DifferentiatorOutMax=[]  FilterDiffOutCoefMin=[]  FilterDiffOutCoefMax=[]  ReciprocalOutMin=[]  ReciprocalOutMax=[]  SumDenOutMin=[]  SumDenOutMax=[]  SumNumOutMin=[]  SumNumOutMax=[]  DivideOutMin=[]  DivideOutMax=[]  UdiffTsProdOutMin=[]  UdiffTsProdOutMax=[]  NTsProdOutMin=[]  NTsProdOutMax=[]  UintegralTsProdOutMin=[]  UintegralTsProdOutMax=[]  UngainTsProdOutMin=[]  UngainTsProdOutMax=[]  ClampingZeroOutDataTypeStr=Inherit: Inherit via back propagation  ClampingZeroOutMin=[]  ClampingZeroOutMax=[]  FilterDenConstantOutDataTypeStr=Inherit: Inherit via back propagation  FilterDenConstantOutMin=[]  FilterDenConstantOutMax=[]  PCopyOutDataTypeStr=Inherit: Inherit via back propagation  PCopyOutMin=[]  PCopyOutMax=[]  NCopyOutDataTypeStr=Inherit: Inherit via back propagation  NCopyOutMin=[]  NCopyOutMax=[]  IntegratorContinuousStateAttributes=''  IntegratorStateMustResolveToSignalObject=off  IntegratorRTWStateStorageClass=Auto  FilterContinuousStateAttributes=''  FilterStateMustResolveToSignalObject=off  FilterRTWStateStorageClass=Auto  ParallelPVariant=InternalParameters  IdealPVariant=Disabled  IVariant=InternalParameters  DVariant=Disabled  IntegratorVariant=Continuous  SatVariant=Disabled  AWVariant=Passthrough  PCopyVariant=Disabled  TRVariant=Disabled  FdbkBlocksVariant=Forward  IdealPFdbkVariant=Disabled  SatFdbkVariant=Disabled  DerivativeFilterVariant=Disabled  NVariant=Disabled  NCopyVariant=Disabled_SignalSpec  FilterICVariant=Disabled  IntegratorICVariant=InternalICs  ExternalResetVariant=Disabled  TRSumVariant=Passthrough  SumFdbkVariant=Disabled  SumVariant=Sum_PI  TsampFilterVariant=InternalTs  TsampNgainVariant=Passthrough  TsampIntegralVariant=Disabled_SignalSpec  ExternalSaturationOutDataTypeStr=Inherit: Same as second input  DerivativeSourceVariant=Disabled  PreIntVariant=InternalPreInt
  Pstep : Step  Time=0.01  After=Pref  SampleTime=0
  Qstep : Step  Time=0.01  After=Qref  SampleTime=0
  Step : Step  Time=0.2  After=2e6  SampleTime=0
  iref : Outport
  PQrefs : Outport  Port=2
  wires:
  Pstep/1 -> Add/1, Mux1/1  "Pref"
  PQ/1 -> Demux1/1
  Mux/1 -> iref/1
  Mux1/1 -> PQrefs/1
  Demux1/1 -> Add/2  "Pmeas"
  Demux1/2 -> Add1/1  "Qmeas"
  Add/1 -> PID Controller/1
  Add1/1 -> PID Controller1/1
  PID Controller1/1 -> Mux/2
  PID Controller/1 -> Mux/1
  Qstep/1 -> Add2/1  "Qref"
  Step/1 -> Add2/2
  Add2/1 -> Mux1/2, Add1/2  "Qref"

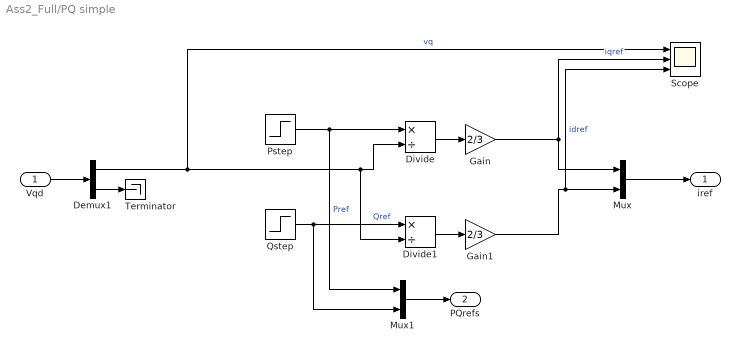
== system Ass2_Full/PQ simple ==
  Vqd : Inport
  Demux1 : Demux  Outputs=2
  Divide : Product  Inputs=*/
  Divide1 : Product  Inputs=*/
  Gain : Gain  Gain=2/3
  Gain1 : Gain  Gain=2/3
  Mux : Mux  Inputs=2
  Mux1 : Mux  Inputs=2
  Pstep : Step  Time=0.01  After=Pref  SampleTime=0
  Qstep : Step  Time=0.01  After=Qref  SampleTime=0
  Scope : Scope  NumInputPorts=3
  Terminator : Terminator
  iref : Outport
  PQrefs : Outport  Port=2
  wires:
  Pstep/1 -> Mux1/1, Divide/1  "Pref"
  Gain1/1 -> Scope/3, Mux/2  "idref"
  Divide1/1 -> Gain1/1
  Qstep/1 -> Mux1/2, Divide1/1  "Qref"
  Demux1/2 -> Terminator/1
  Demux1/1 -> Scope/1, Divide1/2, Divide/2  "vq"
  Vqd/1 -> Demux1/1
  Divide/1 -> Gain/1
  Gain/1 -> Mux/1, Scope/2  "iqref"
  Mux/1 -> iref/1
  Mux1/1 -> PQrefs/1

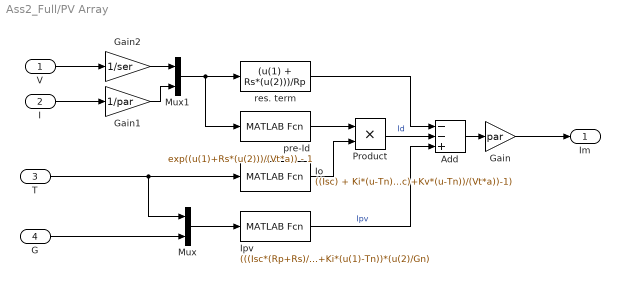
== system Ass2_Full/PV Array ==
  V : Inport
  I : Inport  Port=2
  T : Inport  Port=3
  G : Inport  Port=4
  Add : Sum  Inputs=--+
  Gain : Gain  Gain=par
  Gain1 : Gain  Gain=1/par
  Gain2 : Gain  Gain=1/ser
  Io : MATLABFcn  MATLABFcn=((Isc) + Ki*(u-Tn)) / ( exp(((Voc)+Kv*(u-Tn))/(Vt*a))-1)
  Ipv : MATLABFcn  MATLABFcn=(((Isc*(Rp+Rs)/Rp))+Ki*(u(1)-Tn))*(u(2)/Gn)
  Mux : Mux  Inputs=2
  Mux1 : Mux  Inputs=2
  Product : Product
  pre-Id : MATLABFcn  MATLABFcn=exp((u(1)+Rs*(u(2)))/(Vt*a)) - 1
  res. term : MATLABFcn  MATLABFcn=(u(1) + Rs*(u(2)))/Rp
  Im : Outport
  wires:
  G/1 -> Mux/2
  res. term/1 -> Add/1
  pre-Id/1 -> Product/1
  Mux/1 -> Ipv/1
  Ipv/1 -> Add/3  "Ipv"
  Mux1/1 -> pre-Id/1, res. term/1
  Gain/1 -> Im/1
  Product/1 -> Add/2  "Id"
  Io/1 -> Product/2
  Add/1 -> Gain/1
  T/1 -> Mux/1, Io/1
  Gain2/1 -> Mux1/1
  Gain1/1 -> Mux1/2
  I/1 -> Gain1/1
  V/1 -> Gain2/1

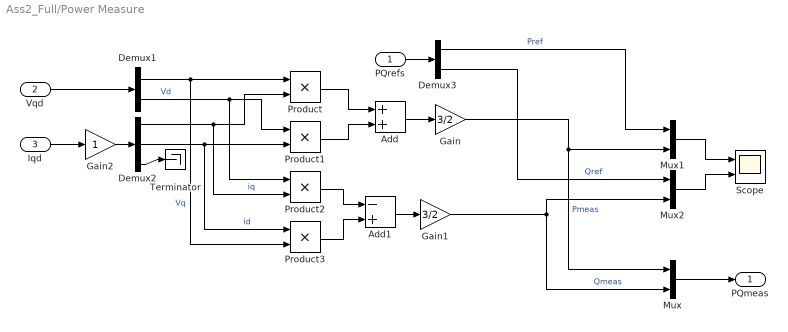
== system Ass2_Full/Power Measure ==
  PQrefs : Inport
  Vqd : Inport  Port=2
  Iqd : Inport  Port=3
  Add : Sum
  Add1 : Sum  Inputs=-+
  Demux1 : Demux  Outputs=2
  Demux2 : Demux  Outputs=3
  Demux3 : Demux  Outputs=2
  Gain : Gain  Gain=3/2
  Gain1 : Gain  Gain=3/2
  Gain2 : Gain
  Mux : Mux  Inputs=2
  Mux1 : Mux  Inputs=2
  Mux2 : Mux  Inputs=2
  Product{,1..3} (4 alike) : Product
  Scope : Scope  NumInputPorts=2
  Terminator : Terminator
  PQmeas : Outport
  wires:
  Product/1 -> Add/1
  PQrefs/1 -> Demux3/1
  Demux2/1 -> Product/2, Product2/2  "iq"
  Vqd/1 -> Demux1/1
  Gain1/1 -> Mux2/2, Mux/2  "Qmeas"
  Demux2/2 -> Product3/1, Product1/2  "id"
  Add/1 -> Gain/1
  Product3/1 -> Add1/2
  Demux3/2 -> Mux2/1  "Qref"
  Product1/1 -> Add/2
  Iqd/1 -> Gain2/1
  Demux1/2 -> Product2/1, Product1/1  "Vd"
  Demux1/1 -> Product3/2, Product/1  "Vq"
  Gain/1 -> Mux1/2, Mux/1  "Pmeas"
  Demux3/1 -> Mux1/1  "Pref"
  Add1/1 -> Gain1/1
  Product2/1 -> Add1/1
  Demux2/3 -> Terminator/1
  Gain2/1 -> Demux2/1
  Mux/1 -> PQmeas/1
  Mux1/1 -> Scope/1
  Mux2/1 -> Scope/2

== system Ass2_Full/VSC DC ==
  Controlled Current Source1 : spsControlledCurrentSourceLib/Controlled Current Source  Initialize=on  Source_Type=AC  Amplitude=0  Phase=0  Frequency=0  Measurements=None
  Current Measurement : spsCurrentMeasurementLib/Current Measurement  PhasorSimulation=off  OutputType=Complex  PSBequivalent=0
  Product : Product
  Product1 : Product  Inputs=*/
  Scope : Scope
  Series RLC Branch : spsSeriesRLCBranchLib/Series RLC Branch  LConnTagsString=__new0  RConnTagsString=__new0  BranchType=C  Resistance=1  Inductance=1e-3  SetiL0=off  InitialCurrent=0  Capacitance=Cdc  Setx0=on  InitialVoltage=Vdc_ref  Measurements=None
  Sum of Elements : Sum  Inputs=+
  Voltage Measurement3 : spsVoltageMeasurementLib/Voltage Measurement  PhasorSimulation=off  OutputType=Complex  PSBequivalent=0
  DC + : PMIOPort  Side=Right
  DC - : PMIOPort  Port=2  Side=Right
  Idc : Outport
  Vdc : Outport  Port=2
  wires:
  [vg_abc] -> Product/2
  Product1/1 -> Controlled Current Source1/1
  Sum of Elements/1 -> Product1/1
  Voltage Measurement3/1 -> Vdc/1, Product1/2  "Vdc"
  [ic_abc] -> Product/1
  Product/1 -> Scope/1, Sum of Elements/1
  Current Measurement/1 -> Idc/1
  connections:
  Series RLC Branch/LConn1 -- Current Measurement/RConn1 -- Voltage Measurement3/LConn1 -- Controlled Current Source1/LConn1
  Controlled Current Source1/RConn1 -- Voltage Measurement3/LConn2 -- DC -/RConn1 -- Series RLC Branch/RConn1
  Current Measurement/LConn1 -- DC +/RConn1

== system Ass2_Full/manual iref ==
  Gain : Gain  Gain=iqref
  Gain1 : Gain  Gain=idref
  Mux1 : Mux  Inputs=2
  Step : Step  Time=0.2  SampleTime=0
  Step1 : Step  Time=0.4  SampleTime=0
  iref : Outport
  wires:
  Gain/1 -> Mux1/1
  Step1/1 -> Gain1/1
  Step/1 -> Gain/1
  Gain1/1 -> Mux1/2
  Mux1/1 -> iref/1

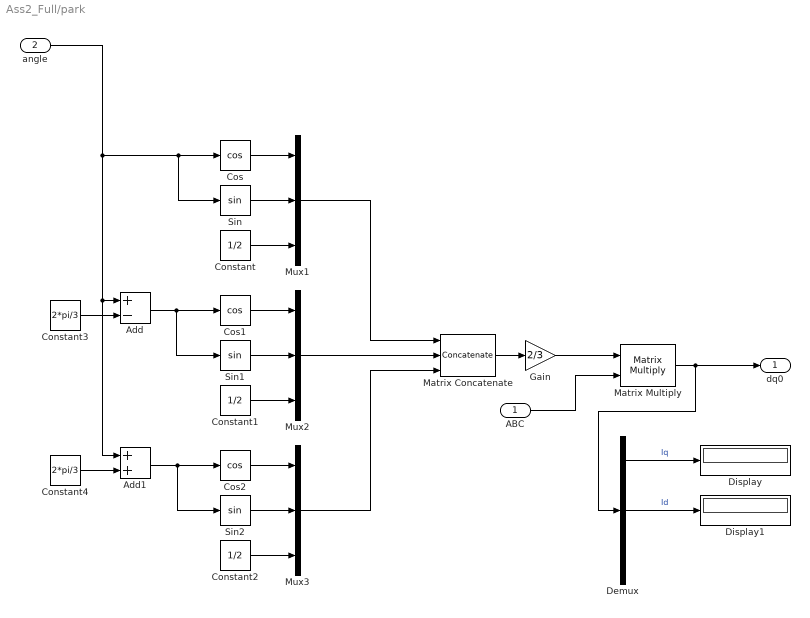
== system Ass2_Full/park ==
  ABC : Inport
  angle : Inport  Port=2
  Add : Sum  Inputs=+-
  Add1 : Sum
  Constant : Constant  Value=1/2
  Constant1 : Constant  Value=1/2
  Constant2 : Constant  Value=1/2
  Constant3 : Constant  Value=2*pi/3
  Constant4 : Constant  Value=2*pi/3
  Cos : Trigonometry  Operator=cos
  Cos1 : Trigonometry  Operator=cos
  Cos2 : Trigonometry  Operator=cos
  Demux : Demux  Outputs=3
  Display : Display
  Display1 : Display
  Gain : Gain  Gain=2/3
  Matrix Concatenate : Concatenate  NumInputs=3  Mode=Multidimensional array  ConcatenateDimension=2
  Matrix Multiply : Product  Multiplication=Matrix(*)
  Mux1 : Mux  Inputs=3
  Mux2 : Mux  Inputs=3
  Mux3 : Mux  Inputs=3
  Sin : Trigonometry
  Sin1 : Trigonometry
  Sin2 : Trigonometry
  dq0 : Outport
  wires:
  Mux2/1 -> Matrix Concatenate/2
  Add/1 -> Sin1/1, Cos1/1
  Add1/1 -> Sin2/1, Cos2/1
  Constant3/1 -> Add/2
  Mux3/1 -> Matrix Concatenate/3
  Gain/1 -> Matrix Multiply/1
  angle/1 -> Add1/1, Add/1, Sin/1, Cos/1
  Cos/1 -> Mux1/1
  Matrix Concatenate/1 -> Gain/1
  Sin/1 -> Mux1/2
  Constant/1 -> Mux1/3
  Sin2/1 -> Mux3/2
  Mux1/1 -> Matrix Concatenate/1
  Cos2/1 -> Mux3/1
  Constant2/1 -> Mux3/3
  Sin1/1 -> Mux2/2
  Cos1/1 -> Mux2/1
  Constant1/1 -> Mux2/3
  Constant4/1 -> Add1/2
  ABC/1 -> Matrix Multiply/2
  Matrix Multiply/1 -> Demux/1, dq0/1
  Demux/1 -> Display/1  "Iq"
  Demux/2 -> Display1/1  "Id"

== system Ass2_Full/Current Loop/inv park ==
  qd0 : Inport
  angle : Inport  Port=2
  Add : Sum  Inputs=+-
  Add1 : Sum
  Constant : Constant
  Constant3 : Constant  Value=2*pi/3
  Constant4 : Constant  Value=2*pi/3
  Cos : Trigonometry  Operator=cos
  Matrix Concatenate : Concatenate  NumInputs=3  Mode=Multidimensional array  ConcatenateDimension=2
  Matrix Multiply : Product  Multiplication=Matrix(*)
  Mux1 : Mux  Inputs=3
  Mux2 : Mux  Inputs=3
  Sin : Trigonometry
  ABC : Outport
  wires:
  Mux2/1 -> Matrix Concatenate/3
  Sin/1 -> Matrix Concatenate/2
  Mux1/1 -> Sin/1, Cos/1
  Matrix Concatenate/1 -> Matrix Multiply/1
  Cos/1 -> Matrix Concatenate/1
  Constant/1 -> Mux2/3, Mux2/1, Mux2/2
  angle/1 -> Add1/1, Mux1/1, Add/1
  Constant4/1 -> Add1/2
  Constant3/1 -> Add/2
  Add/1 -> Mux1/2
  Matrix Multiply/1 -> ABC/1
  qd0/1 -> Matrix Multiply/2
  Add1/1 -> Mux1/3

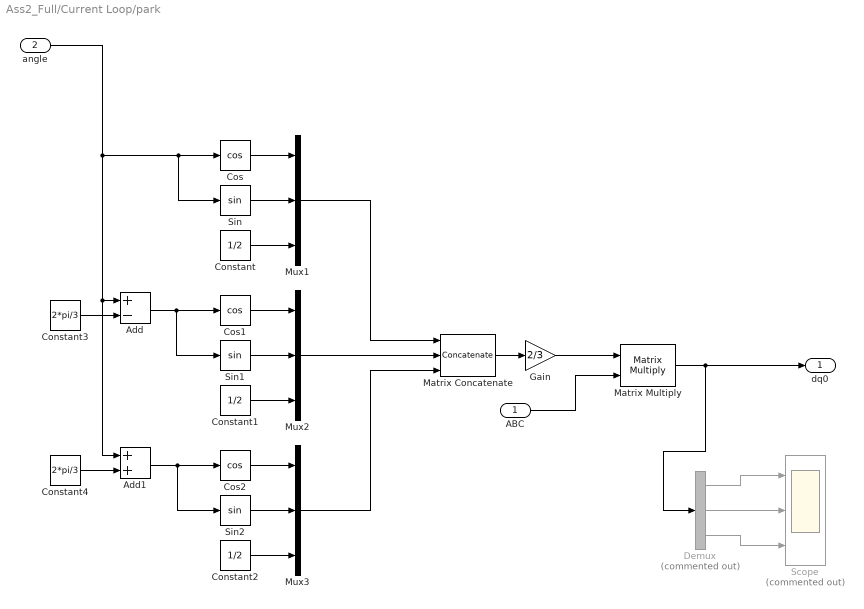
== system Ass2_Full/Current Loop/park ==
  ABC : Inport
  angle : Inport  Port=2
  Add : Sum  Inputs=+-
  Add1 : Sum
  Constant : Constant  Value=1/2
  Constant1 : Constant  Value=1/2
  Constant2 : Constant  Value=1/2
  Constant3 : Constant  Value=2*pi/3
  Constant4 : Constant  Value=2*pi/3
  Cos : Trigonometry  Operator=cos
  Cos1 : Trigonometry  Operator=cos
  Cos2 : Trigonometry  Operator=cos
  Demux : Demux  Commented=on  Outputs=3
  Gain : Gain  Gain=2/3
  Matrix Concatenate : Concatenate  NumInputs=3  Mode=Multidimensional array  ConcatenateDimension=2
  Matrix Multiply : Product  Multiplication=Matrix(*)
  Mux1 : Mux  Inputs=3
  Mux2 : Mux  Inputs=3
  Mux3 : Mux  Inputs=3
  Scope : Scope  Commented=on  NumInputPorts=3
  Sin : Trigonometry
  Sin1 : Trigonometry
  Sin2 : Trigonometry
  dq0 : Outport
  wires:
  Mux2/1 -> Matrix Concatenate/2
  Add/1 -> Sin1/1, Cos1/1
  Add1/1 -> Sin2/1, Cos2/1
  Constant3/1 -> Add/2
  Mux3/1 -> Matrix Concatenate/3
  Gain/1 -> Matrix Multiply/1
  angle/1 -> Add1/1, Add/1, Sin/1, Cos/1
  Cos/1 -> Mux1/1
  Matrix Concatenate/1 -> Gain/1
  Sin/1 -> Mux1/2
  Constant/1 -> Mux1/3
  Sin2/1 -> Mux3/2
  Mux1/1 -> Matrix Concatenate/1
  Cos2/1 -> Mux3/1
  Constant2/1 -> Mux3/3
  Sin1/1 -> Mux2/2
  Cos1/1 -> Mux2/1
  Constant1/1 -> Mux2/3
  Constant4/1 -> Add1/2
  ABC/1 -> Matrix Multiply/2
  Matrix Multiply/1 -> Demux/1, dq0/1
  Demux/1 -> Scope/1
  Demux/2 -> Scope/2
  Demux/3 -> Scope/3

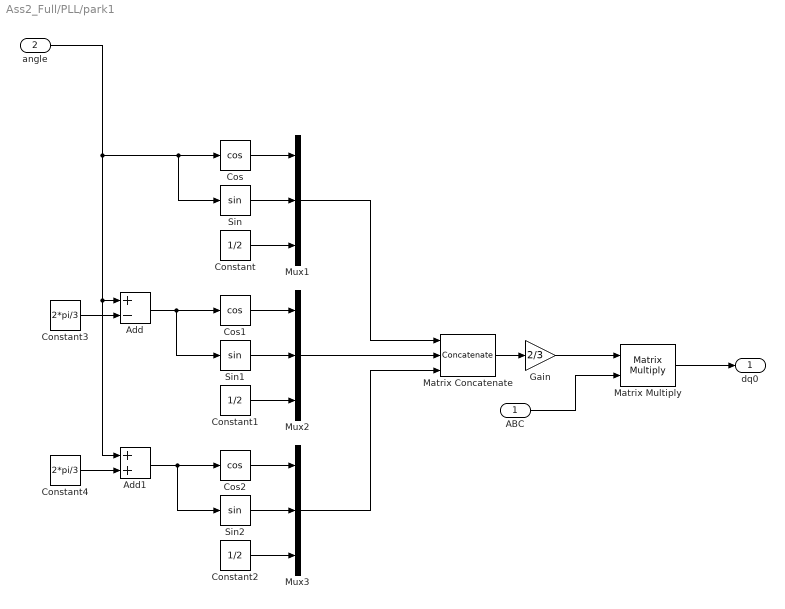
== system Ass2_Full/PLL/park1 ==
  ABC : Inport
  angle : Inport  Port=2
  Add : Sum  Inputs=+-
  Add1 : Sum
  Constant : Constant  Value=1/2
  Constant1 : Constant  Value=1/2
  Constant2 : Constant  Value=1/2
  Constant3 : Constant  Value=2*pi/3
  Constant4 : Constant  Value=2*pi/3
  Cos : Trigonometry  Operator=cos
  Cos1 : Trigonometry  Operator=cos
  Cos2 : Trigonometry  Operator=cos
  Gain : Gain  Gain=2/3
  Matrix Concatenate : Concatenate  NumInputs=3  Mode=Multidimensional array  ConcatenateDimension=2
  Matrix Multiply : Product  Multiplication=Matrix(*)
  Mux1 : Mux  Inputs=3
  Mux2 : Mux  Inputs=3
  Mux3 : Mux  Inputs=3
  Sin : Trigonometry
  Sin1 : Trigonometry
  Sin2 : Trigonometry
  dq0 : Outport
  wires:
  Mux2/1 -> Matrix Concatenate/2
  Add/1 -> Sin1/1, Cos1/1
  Add1/1 -> Sin2/1, Cos2/1
  Constant3/1 -> Add/2
  Mux3/1 -> Matrix Concatenate/3
  Gain/1 -> Matrix Multiply/1
  angle/1 -> Add1/1, Add/1, Sin/1, Cos/1
  Cos/1 -> Mux1/1
  Matrix Concatenate/1 -> Gain/1
  Sin/1 -> Mux1/2
  Constant/1 -> Mux1/3
  Sin2/1 -> Mux3/2
  Mux1/1 -> Matrix Concatenate/1
  Cos2/1 -> Mux3/1
  Constant2/1 -> Mux3/3
  Sin1/1 -> Mux2/2
  Cos1/1 -> Mux2/1
  Constant1/1 -> Mux2/3
  Constant4/1 -> Add1/2
  ABC/1 -> Matrix Multiply/2
  Matrix Multiply/1 -> dq0/1
